simulink model "uploadthreephase"  (R2016a)
settings: Solver=VariableStepAuto  StartTime=0.0  StopTime=60e-3  RelTol=1e-3
libraries: powerlib x23
settings Model: Creator=VARUN SINGH  LastModifiedBy=VARUN SINGH

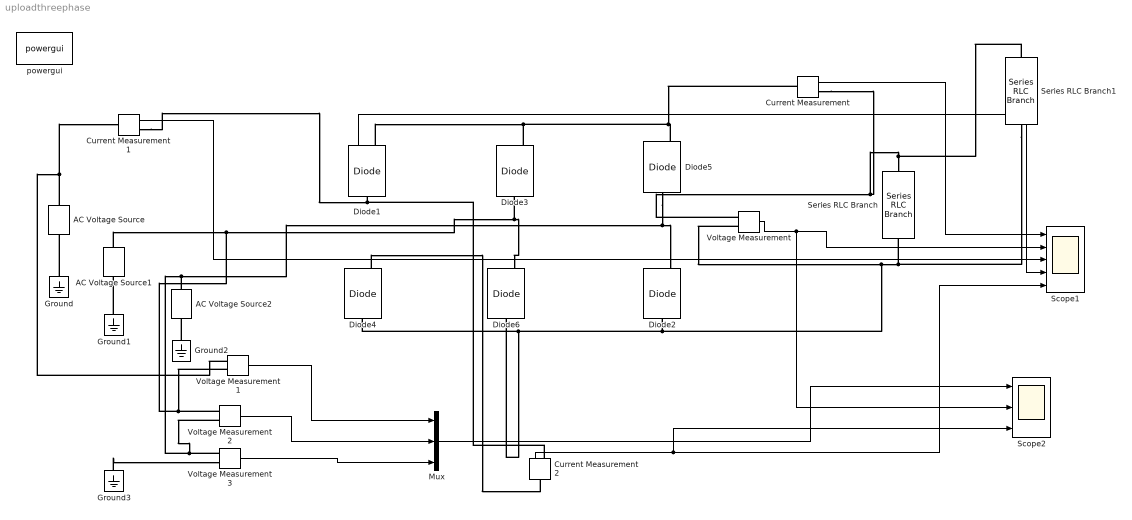
== system uploadthreephase ==
  AC Voltage Source : powerlib/Electrical Sources/AC Voltage Source  Amplitude=230  Phase=0  Frequency=50  SampleTime=0  Measurements=None  BusType=swing  Pref=10e3  Qref=0  Qmin=-inf  Qmax=+inf
  AC Voltage Source1 : powerlib/Electrical Sources/AC Voltage Source  Amplitude=230  Phase=-120  Frequency=50  SampleTime=0  Measurements=None  BusType=swing  Pref=10e3  Qref=0  Qmin=-inf  Qmax=+inf
  AC Voltage Source2 : powerlib/Electrical Sources/AC Voltage Source  Amplitude=230  Phase=-240  Frequency=50  SampleTime=0  Measurements=None  BusType=swing  Pref=10e3  Qref=0  Qmin=-inf  Qmax=+inf
  Current Measurement : powerlib/Measurements/Current Measurement  PhasorSimulation=off  OutputType=Complex  PSBequivalent=0
  Current Measurement1 : powerlib/Measurements/Current Measurement  PhasorSimulation=off  OutputType=Complex  PSBequivalent=0
  Current Measurement2 : powerlib/Measurements/Current Measurement  PhasorSimulation=off  OutputType=Complex  PSBequivalent=0
  Diode{1..6} (6 alike) : powerlib/Power Electronics/Diode  Ron=0.001  Lon=0  Vf=0.8  IC=0  UseSnubber=off  Rs=500  Cs=250e-9  Measurements=on
  Ground{,1..3} (4 alike) : powerlib/Elements/Ground  LConnTagsString=a
  Mux : Mux  Inputs=3
  Scope1 : Scope  NumInputPorts=5
  Scope2 : Scope  NumInputPorts=3
  Series RLC Branch : powerlib/Elements/Series RLC Branch  LConnTagsString=__new0  RConnTagsString=__new0  BranchType=R  Resistance=1  Inductance=1e-3  SetiL0=off  InitialCurrent=0  Capacitance=1e-6  Setx0=off  InitialVoltage=0  Measurements=None
  Series RLC Branch1 : powerlib/Elements/Series RLC Branch  LConnTagsString=__new0  RConnTagsString=__new0  BranchType=C  Resistance=1  Inductance=1e-3  SetiL0=off  InitialCurrent=0  Capacitance=1e-6  Setx0=off  InitialVoltage=0  Measurements=None
  Voltage Measurement{,1..3} (4 alike) : powerlib/Measurements/Voltage Measurement  PhasorSimulation=off  OutputType=Complex  PSBequivalent=0
  powergui : powerlib/powergui  Priority=1  SimulationMode=Continuous  SolverType=Tustin/Backward Euler (TBE)  SampleTime=50e-6  frequency=60  SPID=off  DisableSnubberDevices=off  DisableRonSwitches=off  DisableVfSwitches=off  SwTol=0  DisplayEquations=off  Interpol=off  ExternalGateDelay=off  methode=off  Ts=10  FunctionMessages=off  echomessages=off  HookPort=off  EnableUseOfTLC=off  x0status=blocks  frequencyindice=50  Pbase=100e6  ErrMax=1e-4  Iterations=50  UnitsV=kV  UnitsW=MW  buscounter=0  RestoreLinks=warning  ResistiveCurrentMeasurement=off  Frange=[0:2:500]  Ylog=off  Xlog=on  ShowGrid=off  save=off  variable=ZData  structure=0  ZoomFFT=off  StartTime=0.0  cycles=1  DisplayStyle=1  fundamental=60  FreqAxis=off  MaxFrequency=1000  frequencyindicesteady=1  RmsSteady=1  display=off
  wires:
  Current Measurement/1 -> Scope1/1
  Voltage Measurement/1 -> Scope2/2, Scope1/2
  Current Measurement1/1 -> Scope1/3
  Voltage Measurement1/1 -> Mux/1
  Voltage Measurement2/1 -> Mux/2
  Voltage Measurement3/1 -> Mux/3
  Mux/1 -> Scope2/1
  Current Measurement2/1 -> Scope2/3, Scope1/5
  Diode1/1 -> Scope1/4
  connections:
  Voltage Measurement1/LConn2 -- Voltage Measurement2/LConn1 -- AC Voltage Source1/RConn1 -- Diode6/RConn1 -- Diode3/LConn1
  Current Measurement/LConn1 -- Diode5/RConn1 -- Diode3/RConn1 -- Diode1/RConn1
  Voltage Measurement/LConn2 -- Series RLC Branch1/LConn1 -- Series RLC Branch/LConn1 -- Diode2/LConn1 -- Diode6/LConn1 -- Diode4/LConn1
  Voltage Measurement3/LConn1 -- Voltage Measurement2/LConn2 -- AC Voltage Source2/RConn1 -- Diode2/RConn1 -- Diode5/LConn1
  Current Measurement2/RConn1 -- Current Measurement1/RConn1 -- Diode1/LConn1
  Voltage Measurement1/LConn1 -- AC Voltage Source/RConn1 -- Current Measurement1/LConn1
  Diode4/RConn1 -- Current Measurement2/LConn1
  Ground2/LConn1 -- AC Voltage Source2/LConn1
  Ground/LConn1 -- AC Voltage Source/LConn1
  Ground3/LConn1 -- Voltage Measurement3/LConn2
  Ground1/LConn1 -- AC Voltage Source1/LConn1
  Voltage Measurement/LConn1 -- Current Measurement/RConn1 -- Series RLC Branch1/RConn1 -- Series RLC Branch/RConn1
